simulink model "lung_mecha_extended"  (R2022a)
settings: Solver=odeN  StartTime=0.0  StopTime=10.0  MaxStep=0.01  RelTol=1e-3
model workspace: external: MATLAB File C:\Users\bigba\Dropbox\Uni\MSSF\notes\class notes\Lezione02\lung_mech_extend_parameters.m (data not in the file)
values from neighbouring files (symbols this model uses):
  CL = 0.2    [lung_mech_extend_parameters.m]
  Cs = 0.005    [lung_mech_extend_parameters.m]
  Cw = 0.2    [lung_mech_extend_parameters.m]
  Rc = 1    [lung_mech_extend_parameters.m]
  Rp = 0.5    [lung_mech_extend_parameters.m]
settings Model: Creator=bigba  LastModifiedBy=bigba
settings DebuggingCC: UnconnectedInputMsg=warning  UnconnectedOutputMsg=warning  UnconnectedLineMsg=warning
settings RTWCC: DLArmComputeVersion=19.05

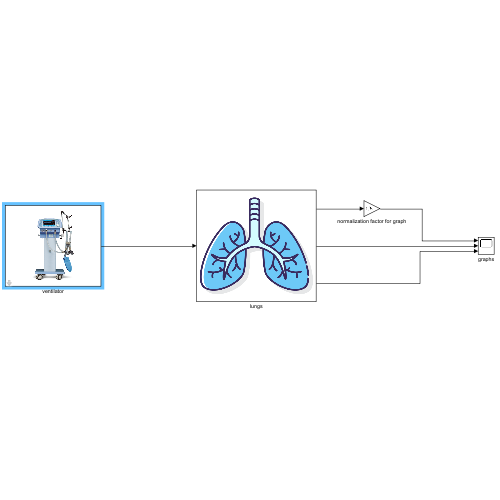
[thumbnail: Simulink's stored preview of the top-level diagram]
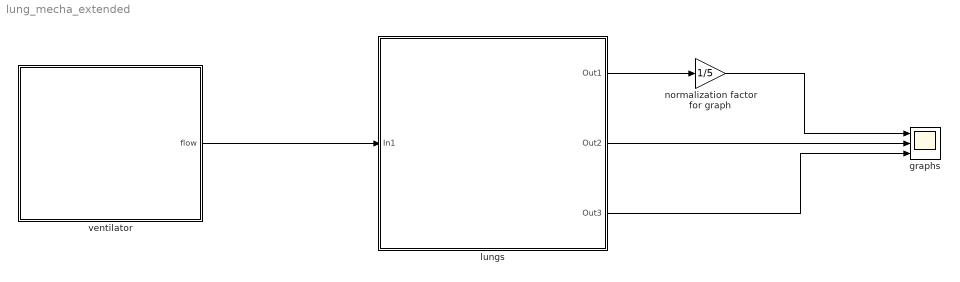
== system lung_mecha_extended ==
  graphs : Scope  NumInputPorts=3
  lungs : Subsystem
      mask Display: image('$imagefile'); % Use "Edit Image" on toolstrip to change.
  normalization factor for graph : Gain  Gain=1/5
  ventilator : Subsystem  mask{breath_for_minute=18, flag_ventilation=1}
      mask TypeOptions flag_ventilation: 1 | 2 | 3
      mask DialogControl Container2 Prompt: Frequency selector
      mask DialogControl Control4 Prompt: Standard: 18 breath/min
      mask DialogControl Control3 Prompt: Set respiratory frequency (breath for minute)
      mask DialogControl Container1 Prompt: Wave type
      mask DialogControl Control2 Prompt: Set:
      mask DialogControl Control7 Prompt: 1 for sine wave;
      mask DialogControl Control5 Prompt: 2 for square wave;
      mask DialogControl Control6 Prompt: 3 for square wave with raise time
      mask Display: image('$imagefile'); % Use "Edit Image" on toolstrip to change.
  wires:
  normalization factor for graph/1 -> graphs/1
  lungs/1(Out1) -> normalization factor for graph/1
  lungs/2(Out2) -> graphs/2
  lungs/3(Out3) -> graphs/3
  ventilator/1(flow) -> lungs/1(In1)

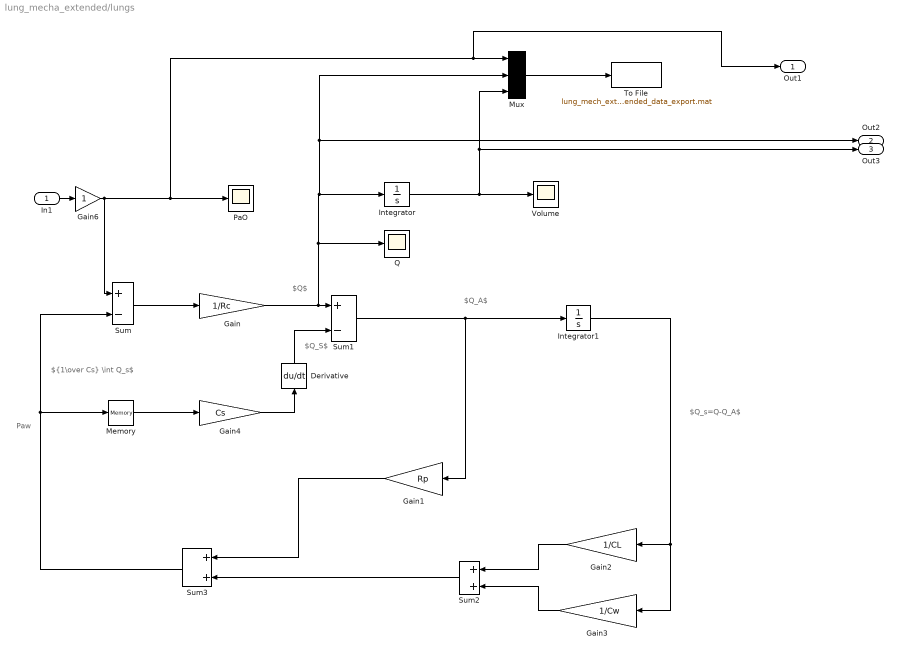
== system lung_mecha_extended/lungs ==
  note: $Q_A$
  note: $Q_s=Q-Q_A$
  note: ${1\over Cs} \int Q_s$
  note: Paw
  note: $Q_S$
  note: $Q$
  In1 : Inport
  Derivative : Derivative
  Gain : Gain  Gain=1/Rc
  Gain1 : Gain  Gain=Rp
  Gain2 : Gain  Gain=1/CL
  Gain3 : Gain  Gain=1/Cw
  Gain4 : Gain  Gain=Cs
  Gain6 : Gain
  Integrator : Integrator
  Integrator1 : Integrator
  Memory : Memory
  Mux : Mux  Inputs=3
  PaO : Scope
  Q : Scope
  Sum : Sum  Inputs=+-
  Sum1 : Sum  Inputs=+-
  Sum2 : Sum
  Sum3 : Sum
  To File : ToFile  Filename=lung_mech_extended_data_export.mat  MatrixName=mechanics_lung  SaveFormat=Timeseries
  Volume : Scope
  Out1 : Outport
  Out2 : Outport  Port=2
  Out3 : Outport  Port=3
  wires:
  Memory/1 -> Gain4/1
  Sum3/1 -> Memory/1, Sum/2
  Gain/1 -> Integrator/1, Out2/1, Mux/2, Q/1, Sum1/1
  Gain1/1 -> Sum3/1
  Sum2/1 -> Sum3/2
  Gain3/1 -> Sum2/2
  Gain2/1 -> Sum2/1
  Integrator1/1 -> Gain2/1, Gain3/1
  Gain4/1 -> Derivative/1
  Integrator/1 -> Out3/1, Mux/3, Volume/1
  Sum/1 -> Gain/1
  Sum1/1 -> Gain1/1, Integrator1/1
  Mux/1 -> To File/1
  Gain6/1 -> Sum/1, Out1/1, Mux/1, PaO/1
  Derivative/1 -> Sum1/2
  In1/1 -> Gain6/1

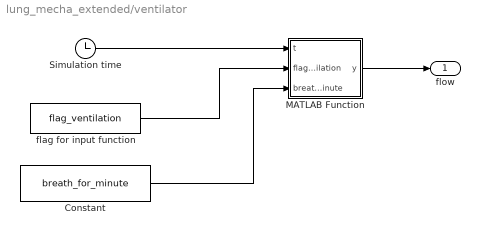
== system lung_mecha_extended/ventilator ==
  Constant : Constant  Value=breath_for_minute
  MATLAB Function : MATLAB Function  TreatAsAtomicUnit=on
  Simulation time : Clock
  flag for input function : Constant  Value=flag_ventilation
  flow : Outport
  wires:
  Simulation time/1 -> MATLAB Function/1(t)
  MATLAB Function/1(y) -> flow/1
  flag for input function/1 -> MATLAB Function/2(flag_ventilation)
  Constant/1 -> MATLAB Function/3(breath_for_minute)

== matlab function lung_mecha_extended/ventilator/MATLAB Function ==
  data: t input; y output; flag_ventilation input; breath_for_minute input
function y = fcn(t,flag_ventilation,breath_for_minute)
% standard conditions: breath_for_minute=18;
f=breath_for_minute/60;
Paw=20;
PEEP=5;
A=0;

% disp(flag_ventilation) %uncomment to debug control variables

if flag_ventilation==1 % flag=1 for sine wave
    A=Paw*sin(2*pi*f*t); % no not use this function, it's also for debugging
    A=PEEP+Paw*sin(2*pi*f*t); % to avoid error use the `odeN` solver !
end

if flag_ventilation==2 % flag=2 for perfect square wave
    tau=0;
    dt=rem(t,(1/f));
    period=1/f;
    half_period=period/2;
    if dt < tau
        A=Paw*(dt/tau)+PEEP;
    end
    if  (dt>=tau) && (dt<half_period)
        A=Paw+PEEP;
    end
    if dt>= (1/f)/2
    A=PEEP;
    end 
end

if flag_ventilation==3 % flag=3 for square wave with raise time tau
    tau=0.35;
    dt=rem(t,(1/f));
    period=1/f;
    half_period=period/2;
    if dt < tau
        A=Paw*(dt/tau)+PEEP;
    end
    if  (dt>=tau) && (dt<half_period)
        A=Paw+PEEP;
    end
    if dt>= (1/f)/2
    A=PEEP;
    end 
end

y=A;

end
